simulink model "mmdlref_conversion_menu_item"  (Simulink 6.3)
settings: Solver=ode5  StartTime=0.0  StopTime=5  FixedStep=0.1  RelTol=1e-3
settings Model: Creator=The MathWorks Inc.  LastModifiedBy=monteiro  ExtModeAutoUpdateStatusClock=off  StrictBusMsg=ErrorLevel1
settings DataIOCC: SignalLoggingName=logsOut
settings OptimizationCC: InlineParams=on  InlineInvariantSignals=on
settings DebuggingCC: CheckExecutionContextPreStartOutputMsg=on  CheckExecutionContextRuntimeOutputMsg=on  SignalResolutionControl=UseLocalSettings  SolverPrmCheckMsg=none  SigSpecEnsureSampleTimeMsg=none
settings HardwareCC: TargetHWDeviceType=32-bit Generic
settings ModelReferenceCC: UpdateModelReferenceTargets=IfOutOfDate
settings RTWCC: ProcessScript=grt_make_rtw_hook
settings CodeAppCC: MaxIdLength=100  CustomSymbolStrFcn=$R$N$F$M  CustomSymbolStrBlkio=rtb_$N$M  CustomSymbolStrType=$N$R$M  CustomSymbolStrLocal=$N$M

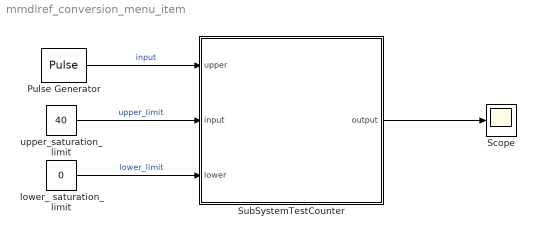
== system mmdlref_conversion_menu_item ==
  Pulse Generator : DiscretePulseGenerator  Amplitude=int32(1)  SampleTime=0.1
  Scope : Scope
      settings: TimeRange=5  YMin=0  YMax=1  DataFormat=Array
  SubSystemTestCounter : Subsystem  TreatAsAtomicUnit=on
  lower_ saturation_ limit : Constant  Value=0  OutDataTypeMode=int32  SampleTime=0.1
  upper_saturation_limit : Constant  Value=40  OutDataTypeMode=int32  SampleTime=0.1
  wires:
  Pulse Generator/1 -> SubSystemTestCounter/1(" upper")  "input"
  upper_saturation_limit/1 -> SubSystemTestCounter/2(" input")  "upper_limit"
  lower_ saturation_ limit/1 -> SubSystemTestCounter/3(lower)  "lower_limit"
  SubSystemTestCounter/1(output) -> Scope/1

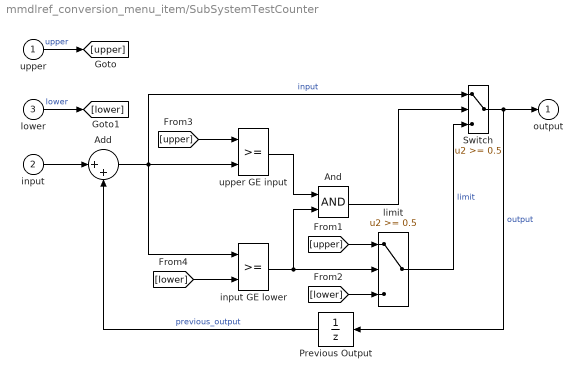
== system mmdlref_conversion_menu_item/SubSystemTestCounter ==
  " upper" : Inport
  " input" : Inport  Port=2
  lower : Inport  Port=3
  " input GE lower" : RelationalOperator  Priority=1  InputSameDT=on
      settings: AttributesFormatString=\n
  " limit" : Switch  Threshold=0.5  SaturateOnIntegerOverflow=on  InputSameDT=on
  Add : Sum  Inputs=|++  OutScaling=2^-10
  And : Logic
  Previous Output : UnitDelay  Orientation=left  SampleTime=-1
  Switch : Switch  Threshold=0.5  SaturateOnIntegerOverflow=on  InputSameDT=on
  upper GE input : RelationalOperator  Priority=0  InputSameDT=on
      settings: AttributesFormatString=\n
  output : Outport
  wires:
  [upper] -> " limit"/1
  Switch/1 -> output/1, Previous Output/1  "output"
  " limit"/1 -> Switch/3  "limit"
  upper GE input/1 -> And/1
  Previous Output/1 -> Add/2  "previous_output"
  " input"/1 -> Add/1
  " upper"/1 -> [upper]  "upper"
  [lower] -> " limit"/3
  [upper] -> upper GE input/1
  [lower] -> " input GE lower"/2
  " input GE lower"/1 -> And/2, " limit"/2
  lower/1 -> [lower]  "lower"
  And/1 -> Switch/2
  Add/1 -> upper GE input/2, " input GE lower"/1, Switch/1  "input"
